simulink model "EB_12B"  (Simulink 8.0)
settings: Solver=ode3  StartTime=0.0  StopTime=0  FixedStep=.01  RelTol=1e-3
undefined symbols (not defined in the file): d, I, I0, up, Wp
settings Model: Creator=elliocm  LastModifiedBy=elliocm
settings DataIOCC: SaveFormat=StructureWithTime  SignalLoggingSaveFormat=ModelDataLogs
settings OptimizationCC: ExpressionDepthLimit=128
settings DebuggingCC: MultiTaskDSMMsg=warning  MultiTaskCondExecSysMsg=none  StateNameClashWarn=none  StrictBusMsg=None
settings RTWCC: IncludeERTFirstTime=on
settings CodeAppCC: CustomSymbolStrType=$N$R$M_T  InternalIdentifier=Shortened

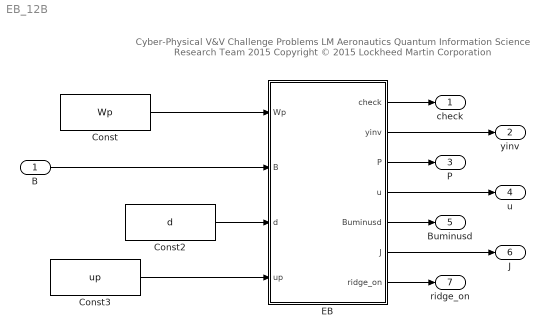
== system EB_12B ==
  note: Cyber-Physical V&V Challenge Problems
      | LM Aeronautics Quantum Information Science Research Team 2015
      | Copyright © 2015 Lockheed Martin Corporation
  B : Inport  OutDataTypeStr=double  PortDimensions=[3 5]
  Const : Constant  Value=Wp
  Const2 : Constant  Value=d
  Const3 : Constant  Value=up
  EB : Subsystem
  check : Outport
  yinv : Outport  Port=2
  P : Outport  Port=3
  u : Outport  Port=4
  Buminusd : Outport  Port=5
  J : Outport  Port=6
  ridge_on : Outport  Port=7
  wires:
  Const/1 -> EB/1(Wp)
  B/1 -> EB/2(B)
  EB/2(yinv) -> yinv/1
  EB/1(check) -> check/1
  Const2/1 -> EB/3(d)
  EB/3(P) -> P/1
  EB/4(u) -> u/1
  Const3/1 -> EB/4(up)
  EB/5(Buminusd) -> Buminusd/1
  EB/6(J) -> J/1
  EB/7(ridge_on) -> ridge_on/1

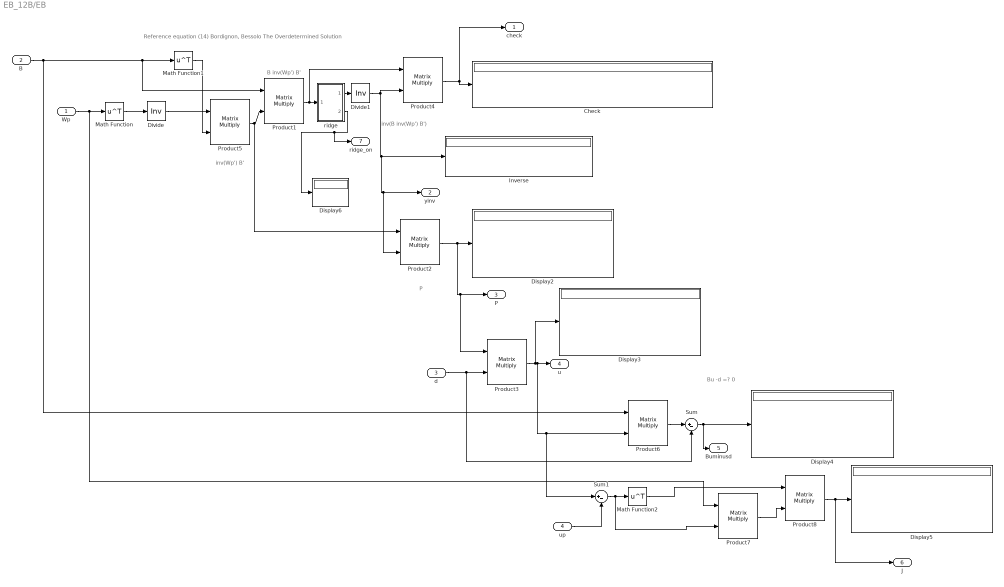
== system EB_12B/EB ==
  note: Reference equation (14) Bordignon, Bessolo
      | The Overdetermined Solution
  note: Bu -d =? 0
  note: P
  note: B inv(Wp') B'
  note: inv(B inv(Wp') B')
  note: inv(Wp') B'
  Wp : Inport
  B : Inport  Port=2
  d : Inport  Port=3
  up : Inport  Port=4
  Check : Display
      settings: Decimation=15
  Display{2..6} (5 alike) : Display
  Divide : Product  Inputs=/  Multiplication=Matrix(*)
  Divide1 : Product  Inputs=/  Multiplication=Matrix(*)
  Inverse : Display
  Math Function : Math  Operator=transpose  SaturateOnIntegerOverflow=on
  Math Function1 : Math  Operator=transpose  SaturateOnIntegerOverflow=on
  Math Function2 : Math  Operator=transpose  SaturateOnIntegerOverflow=on
  Product{1..8} (8 alike) : Product  Multiplication=Matrix(*)
  Sum : Sum  Inputs=|+-
  Sum1 : Sum  Inputs=|+-
  ridge : Subsystem
  check : Outport
  yinv : Outport  Port=2
  P : Outport  Port=3
  u : Outport  Port=4
  Buminusd : Outport  Port=5
  J : Outport  Port=6
  ridge_on : Outport  Port=7
  wires:
  Product1/1 -> Product4/1, ridge/1(In1)
  ridge/1(Out1) -> Divide1/1
  Divide/1 -> Product5/1
  Divide1/1 -> Product2/2, yinv/1, Inverse/1, Product4/2
  Math Function1/1 -> Product5/2
  B/1 -> Product6/1, Product1/1, Math Function1/1
  Math Function/1 -> Divide/1
  Wp/1 -> Product7/1, Math Function/1
  Product5/1 -> Product2/1, Product1/2
  Product4/1 -> check/1, Check/1
  Product2/1 -> Product3/1, P/1, Display2/1
  d/1 -> Sum/2, Product3/2
  Product3/1 -> Display3/1, Sum1/1, Product6/2, u/1
  Product6/1 -> Sum/1
  Sum/1 -> Buminusd/1, Display4/1
  up/1 -> Sum1/2
  Sum1/1 -> Product7/2, Math Function2/1
  Math Function2/1 -> Product8/1
  Product7/1 -> Product8/2
  Product8/1 -> J/1, Display5/1
  ridge/2(ridge_on) -> ridge_on/1, Display6/1

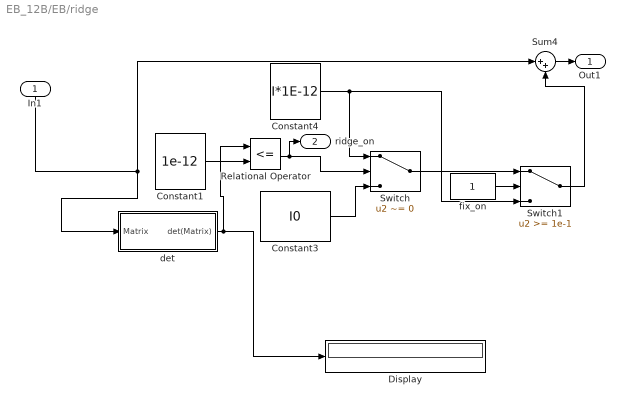
== system EB_12B/EB/ridge ==
  In1 : Inport
  Constant1 : Constant  Value=1e-12
  Constant3 : Constant  Value=I0
  Constant4 : Constant  Value=I*1E-12
  Display : Display
  Relational Operator : RelationalOperator  Operator=<=  OutDataTypeStr=boolean
  Sum4 : Sum  Inputs=|++
  Switch : Switch  Criteria=u2 ~= 0  Threshold=1e-5
  Switch1 : Switch  Threshold=1e-1
  det : Subsystem
  fix_on : Constant
  Out1 : Outport
  ridge_on : Outport  Port=2
  wires:
  Sum4/1 -> Out1/1
  Constant4/1 -> Switch/1, Switch1/3
  In1/1 -> Sum4/1, det/1(Matrix)
  Switch1/1 -> Sum4/2
  Switch/1 -> Switch1/1
  fix_on/1 -> Switch1/2
  det/1(det(Matrix)) -> Relational Operator/1, Display/1
  Relational Operator/1 -> ridge_on/1, Switch/2
  Constant1/1 -> Relational Operator/2
  Constant3/1 -> Switch/3

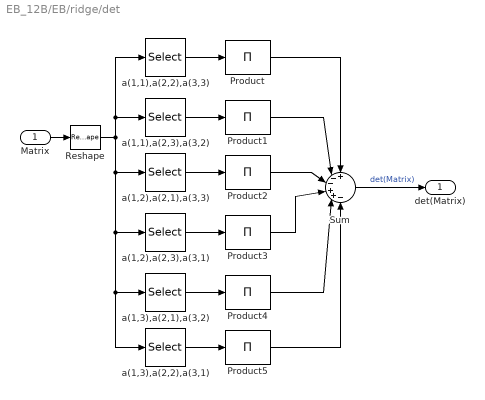
== system EB_12B/EB/ridge/det ==
  Matrix : Inport  PortDimensions=[3 3]
  Product{,1..5} (6 alike) : Product  Inputs=1  SaturateOnIntegerOverflow=on  OutDataTypeStr=Inherit: Same as first input
  Reshape : Reshape  OutputDimensionality=Column vector (2-D)
  Sum : Sum  Inputs=+--++-  SaturateOnIntegerOverflow=on
  a(1,1),a(2,2),a(3,3) : Selector  InputPortWidth=9  IndexOptions=Index vector (dialog)  Indices=[1 5 9]  OutputSizes=1
  a(1,1),a(2,3),a(3,2) : Selector  InputPortWidth=9  IndexOptions=Index vector (dialog)  Indices=[1 6 8]  OutputSizes=1
  a(1,2),a(2,1),a(3,3) : Selector  InputPortWidth=9  IndexOptions=Index vector (dialog)  Indices=[2 4 9]  OutputSizes=1
  a(1,2),a(2,3),a(3,1) : Selector  InputPortWidth=9  IndexOptions=Index vector (dialog)  Indices=[3 4 8]  OutputSizes=1
  a(1,3),a(2,1),a(3,2) : Selector  InputPortWidth=9  IndexOptions=Index vector (dialog)  Indices=[2 6 7]  OutputSizes=1
  a(1,3),a(2,2),a(3,1) : Selector  InputPortWidth=9  IndexOptions=Index vector (dialog)  Indices=[3 5 7]  OutputSizes=1
  det(Matrix) : Outport  PortDimensions=1
  wires:
  a(1,1),a(2,2),a(3,3)/1 -> Product/1
  a(1,1),a(2,3),a(3,2)/1 -> Product1/1
  a(1,2),a(2,1),a(3,3)/1 -> Product2/1
  a(1,2),a(2,3),a(3,1)/1 -> Product3/1
  a(1,3),a(2,1),a(3,2)/1 -> Product4/1
  a(1,3),a(2,2),a(3,1)/1 -> Product5/1
  Product/1 -> Sum/1
  Product1/1 -> Sum/2
  Product2/1 -> Sum/3
  Product3/1 -> Sum/4
  Product4/1 -> Sum/5
  Product5/1 -> Sum/6
  Matrix/1 -> Reshape/1
  Sum/1 -> det(Matrix)/1  "det(Matrix)"
  Reshape/1 -> a(1,1),a(2,2),a(3,3)/1, a(1,1),a(2,3),a(3,2)/1, a(1,2),a(2,1),a(3,3)/1, a(1,2),a(2,3),a(3,1)/1, a(1,3),a(2,1),a(3,2)/1, a(1,3),a(2,2),a(3,1)/1
